simulink library "Power_Shaft1_Ideal_A1"  (R2023a)
settings: Solver=VariableStepAuto  StartTime=0.0  StopTime=10.0  RelTol=1e-3
libraries: fl_lib x2, sm_lib x1, Power_Components x1, nesl_utility x1
Description:
  | Component of Simscape Vehicle Templates Library
  | 
  | Copyright 2018-2024 The MathWorks, Inc.
settings Model: Creator=smiller  LastModifiedBy=smiller
settings SolverCC: AlgebraicLoopSolver=TrustRegion
settings DataIOCC: ReturnWorkspaceOutputs=off
settings DebuggingCC: UnconnectedInputMsg=warning  UnconnectedOutputMsg=warning  UnconnectedLineMsg=warning  ArithmeticOperatorsInVariantConditions=warning
settings ModelReferenceCC: EnableRefExpFcnMdlSchedulingChecks=on
settings SFSimCC: CustomCodeUndefinedFunction=UseInterfaceOnly
settings RTWCC: DLArmComputeVersion=19.05

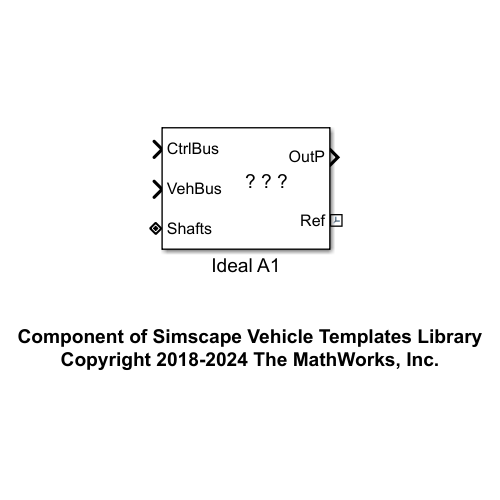
[thumbnail: Simulink's stored preview of the top-level diagram]
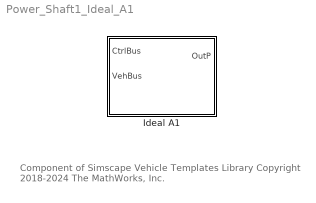
== system Power_Shaft1_Ideal_A1 ==
  note: Component of Simscape Vehicle Templates Library
      | Copyright 2018-2024 The MathWorks, Inc.
  Ideal A1 : Subsystem  VariantControl=IdealOneMotor  mask(Single Ideal Motor, First Axle){motor_ts_f=100}
      mask prompts: motor_ts_f "Motor Axle 1 Cutoff Frequency (Hz)"
      mask help: Models an ideal motor connected to first axle in vehicle driveline.
      mask Display: image('sm_car_vehicle_power_i1motor_A1_IMAGE.png');

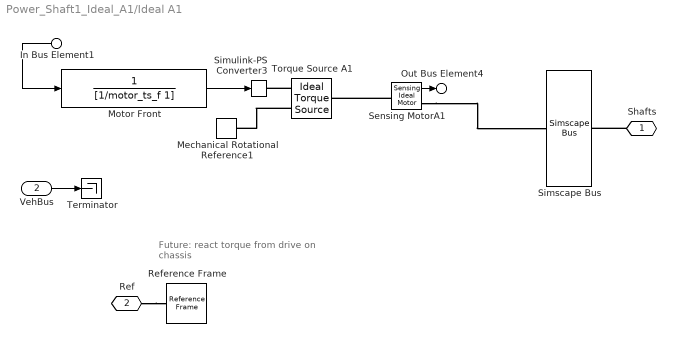
== system Power_Shaft1_Ideal_A1/Ideal A1 ==
  note: Future: react torque from
      | drive on chassis
  In Bus Element1 : Inport  PortName=CtrlBus  Element=MMotorA1Demand
  VehBus : Inport  Port=2
  Mechanical Rotational Reference1 : fl_lib/Mechanical/Rotational Elements/Mechanical Rotational Reference
  Motor Front : TransferFcn  Denominator=[1/motor_ts_f 1]
  Reference Frame : sm_lib/Frames and Transforms/Reference Frame
  Sensing MotorA1 : Power_Components/Sensing Ideal Motor  SystemSampleTime=-1  VariantActivationTime=update diagram  Latency=0  AutoFrameSizeCalculation=off
  Simscape Bus : SimscapeBus  HierarchyStrings=ShaftA1
  Simulink-PS Converter3 : nesl_utility/Simulink-PS Converter  PhysicalDomain=network_engine_domain  SubClassName=ps_input  LeftPortType=input  RightPortType=output  PseudoPeriodic=off  Frequencies=[]  NoiseDistribution=none  NoiseParameters=[]  Unit=1  AffineConversion=off  FilteringAndDerivatives=provide  SimscapeFilterOrder=1  InputFilterTimeConstant=0.001  UdotUserProvided=0
  Terminator : Terminator
  Torque Source A1 : fl_lib/Mechanical/Mechanical Sources/Ideal Torque Source
  Shafts : PMIOPort  Side=Left
  Ref : PMIOPort  Port=2  Side=Right
  Out Bus Element4 : Outport  VectorParamsAs1DForOutWhenUnconnected=off  PortName=OutP  Element=MotorA1
  wires:
  In Bus Element1/1 -> Motor Front/1
  Motor Front/1 -> Simulink-PS Converter3/1
  VehBus/1 -> Terminator/1
  Sensing MotorA1/1 -> Out Bus Element4/1
  connections:
  Sensing MotorA1/LConn1 -- Torque Source A1/LConn1
  Torque Source A1/RConn1 -- Simulink-PS Converter3/RConn1
  Torque Source A1/RConn2 -- Mechanical Rotational Reference1/LConn1
  Shafts/RConn1 -- Simscape Bus/RConn1
  Ref/RConn1 -- Reference Frame/RConn1
  Sensing MotorA1/RConn1 -- Simscape Bus/LConn1
